simulink model "RngMod_TrqFrcCalc"  (R2016b)
settings: configuration reference "CodeGenConfigSet" (kept outside this file)
values from neighbouring files (symbols this model uses):
  RngMod_numTrqFrc_C = Calibration.Parameter    [init_RngMod_TrqFrcCalc.m]
  RngMod_trqFrc_MAP = Calibration.Parameter    [init_RngMod_TrqFrcCalc.m]
  RngMod_trqFrc_MAPX = Calibration.Parameter    [init_RngMod_TrqFrcCalc.m]
  RngMod_trqFrc_MAPY = Calibration.Parameter    [init_RngMod_TrqFrcCalc.m]
  RngMod_trqLossComp_C = Calibration.Parameter    [init_RngMod_TrqFrcCalc.m]
settings Model: Creator=Wollf  LastModifiedBy=wangrui
settings ConfigSetRef: SourceLocation=Base Workspace

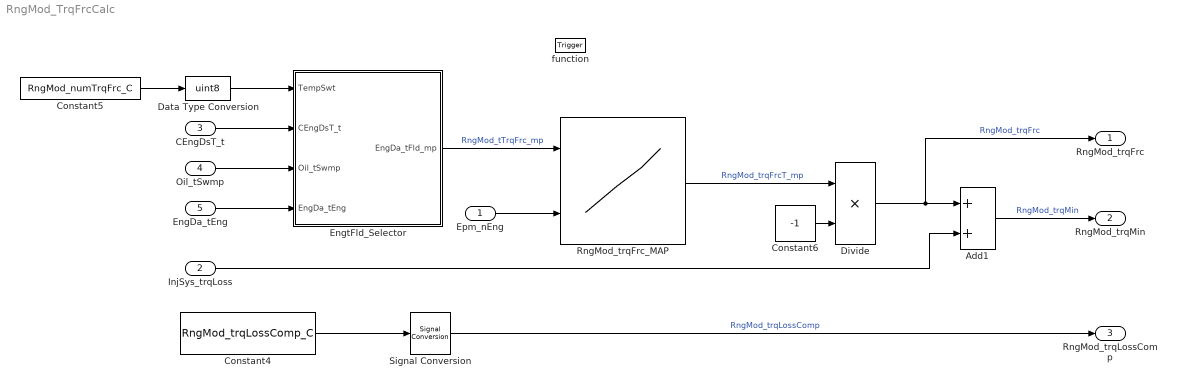
== system RngMod_TrqFrcCalc ==
  Epm_nEng : Inport  Tag=rpm  Description=Engine speed  OutMin=0  OutMax=6000  OutDataTypeStr=EngSpeed_rpm
  InjSys_trqLoss : Inport  Tag=Nm  Description=Torque loss of injection system  Port=2  OutMin=-3276.8  OutMax=3276.7  OutDataTypeStr=Trq_Nm
  CEngDsT_t : Inport  Tag=deg  Description=engine coolant temperature after filter  Port=3  OutMin=-200  OutMax=200  OutDataTypeStr=Temp_deg
  Oil_tSwmp : Inport  Tag=deg  Description=Oil temperature in oil sump  Port=4  OutMin=-50  OutMax=200  OutDataTypeStr=Temp_deg
  EngDa_tEng : Inport  Tag=deg  Description=Engine temperature  Port=5  OutMin=-1000  OutMax=1000  OutDataTypeStr=Temp_deg
  function : TriggerPort  TriggerType=function-call  VariantControl=Variant
  Add1 : Sum  SaturateOnIntegerOverflow=on  InputSameDT=on
  Constant4 : Constant  Value=RngMod_trqLossComp_C  OutDataTypeStr=Inherit: Inherit via back propagation
  Constant5 : Constant  Value=RngMod_numTrqFrc_C
  Constant6 : Constant  Value=-1  OutDataTypeStr=Inherit: Inherit via back propagation
  Data Type Conversion : DataTypeConversion  OutDataTypeStr=uint8
  Divide : Product  Inputs=**  OutDataTypeStr=Trq_Nm
  EngtFld_Selector : Subsystem
  RngMod_trqFrc_MAP : Lookup_n-D  BreakpointsForDimension1=RngMod_trqFrc_MAPY  BreakpointsForDimension2=RngMod_trqFrc_MAPX  IndexSearchMethod=Linear search  BeginIndexSearchUsingPreviousIndexResult=on  Table=RngMod_trqFrc_MAP  ExtrapMethod=Clip  UseLastTableValue=on  InternalRulePriority=Speed  OutDataTypeStr=Inherit: Inherit via back propagation  SaturateOnIntegerOverflow=on
  Signal Conversion : SignalConversion  OverrideOpt=off
  RngMod_trqFrc : Outport  Tag=Nm  Description=Current friction torque  OutMin=-3276.8  OutMax=3276.7  OutDataTypeStr=Trq_Nm
  RngMod_trqMin : Outport  Tag=Nm  Description=Drag torque (minimum torque)  Port=2  OutMin=-3276.8  OutMax=3276.7  OutDataTypeStr=Trq_Nm
  RngMod_trqLossComp : Outport  Tag=Nm  Description=compensation for torque  Port=3  OutMin=-3276.8  OutMax=3276.7  OutDataTypeStr=Trq_Nm
  wires:
  Divide/1 -> RngMod_trqFrc/1, Add1/1  "RngMod_trqFrc"
  InjSys_trqLoss/1 -> Add1/2
  Constant5/1 -> Data Type Conversion/1
  RngMod_trqFrc_MAP/1 -> Divide/1  "RngMod_trqFrcT_mp"
  Epm_nEng/1 -> RngMod_trqFrc_MAP/2
  Constant6/1 -> Divide/2
  EngtFld_Selector/1(EngDa_tFld_mp) -> RngMod_trqFrc_MAP/1  "RngMod_tTrqFrc_mp"
  Add1/1 -> RngMod_trqMin/1  "RngMod_trqMin"
  Constant4/1 -> Signal Conversion/1
  Signal Conversion/1 -> RngMod_trqLossComp/1  "RngMod_trqLossComp"
  Data Type Conversion/1 -> EngtFld_Selector/1(TempSwt)
  CEngDsT_t/1 -> EngtFld_Selector/2(CEngDsT_t)
  Oil_tSwmp/1 -> EngtFld_Selector/3(Oil_tSwmp)
  EngDa_tEng/1 -> EngtFld_Selector/4(EngDa_tEng)

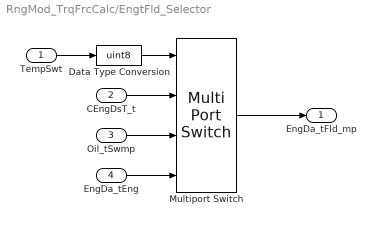
== system RngMod_TrqFrcCalc/EngtFld_Selector ==
  TempSwt : Inport
  CEngDsT_t : Inport  Tag=deg  Description=engine coolant temperature after filter  Port=2
  Oil_tSwmp : Inport  Tag=deg  Description=Oil temperature in oil sump  Port=3
  EngDa_tEng : Inport  Tag=deg  Description=Engine temperature  Port=4
  Data Type Conversion : DataTypeConversion  OutDataTypeStr=uint8
  Multiport Switch : MultiPortSwitch  DataPortOrder=Zero-based contiguous
  EngDa_tFld_mp : Outport  Tag=deg  Description=Engine temperature field
  wires:
  CEngDsT_t/1 -> Multiport Switch/2
  Multiport Switch/1 -> EngDa_tFld_mp/1
  EngDa_tEng/1 -> Multiport Switch/4
  Oil_tSwmp/1 -> Multiport Switch/3
  Data Type Conversion/1 -> Multiport Switch/1
  TempSwt/1 -> Data Type Conversion/1
